simulink model "Buck_ZCS"  (R2024a)
settings: Solver=VariableStepAuto  StartTime=0.0  StopTime=10.0  RelTol=1e-3
values from neighbouring files (symbols this model uses):
  Cr = 10^(-6)    (= 1e-06)    [Parameters.m]
  Fs = 100*10^(3)    (= 100000)    [Parameters.m]
  Io = 1    [Parameters.m]
  Lr = 10*10^(-6)    (= 1e-05)    [Parameters.m]
  R = 7.69    [Parameters.m]
  Vin = 12    [Parameters.m]
  Wo = 1/sqrt(Lr*Cr)    [Parameters.m]
  Zo = sqrt(Lr/Cr)    [Parameters.m]
libraries: spsSeriesRLCBranchLib x6, spsCurrentMeasurementLib x2, spsDiodeLib x2, spsDCVoltageSourceLib x1, spsMosfetLib x1, spsVoltageMeasurementLib x1, sps_lib x1
settings Model: Creator=User  LastModifiedBy=User

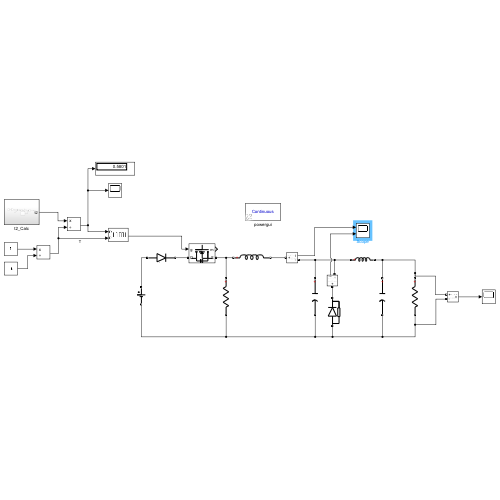
[thumbnail: Simulink's stored preview of the top-level diagram]
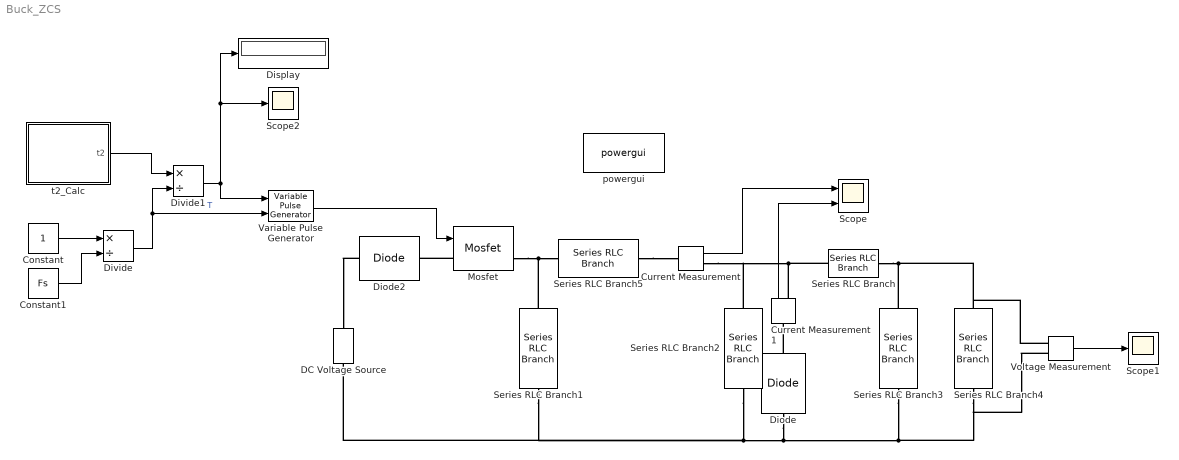
== system Buck_ZCS ==
  Constant : Constant
  Constant1 : Constant  Value=Fs
  Current Measurement : spsCurrentMeasurementLib/Current Measurement  PhasorSimulation=off  OutputType=Complex  PSBequivalent=0
  Current Measurement1 : spsCurrentMeasurementLib/Current Measurement  PhasorSimulation=off  OutputType=Complex  PSBequivalent=0
  DC Voltage Source : spsDCVoltageSourceLib/DC Voltage Source  Amplitude=Vin  Measurements=None
  Diode : spsDiodeLib/Diode  Ron=0.001  Lon=0  Vf=0.8  IC=0  UseSnubber=0  Rs=500  Cs=250e-9  Measurements=off
  Diode2 : spsDiodeLib/Diode  Ron=0.001  Lon=0  Vf=0.8  IC=0  UseSnubber=0  Rs=500  Cs=0  Measurements=off
  Display : Display
  Divide : Product  Inputs=*/
  Divide1 : Product  Inputs=*/
  Mosfet : spsMosfetLib/Mosfet  Ron=0.1  Lon=0  Rd=0.01  Vfd=0  IC=0  Rs=1e5  Cs=inf  Measurements=on
  Scope : Scope  NumInputPorts=2
  Scope1 : Scope
  Scope2 : Scope
  Series RLC Branch : spsSeriesRLCBranchLib/Series RLC Branch  LConnTagsString=__new0  RConnTagsString=__new0  BranchType=L  Resistance=1  Inductance=5e-3  SetiL0=off  InitialCurrent=0  Capacitance=1e-6  Setx0=off  InitialVoltage=0  Measurements=None
  Series RLC Branch1 : spsSeriesRLCBranchLib/Series RLC Branch  LConnTagsString=__new0  RConnTagsString=__new0  BranchType=R  Resistance=10000  Inductance=1e-3  SetiL0=off  InitialCurrent=0  Capacitance=1e-6  Setx0=off  InitialVoltage=0  Measurements=None
  Series RLC Branch2 : spsSeriesRLCBranchLib/Series RLC Branch  LConnTagsString=__new0  RConnTagsString=__new0  BranchType=C  Resistance=1  Inductance=1e-3  SetiL0=off  InitialCurrent=0  Capacitance=Cr  Setx0=off  InitialVoltage=0  Measurements=None
  Series RLC Branch3 : spsSeriesRLCBranchLib/Series RLC Branch  LConnTagsString=__new0  RConnTagsString=__new0  BranchType=C  Resistance=1  Inductance=1e-3  SetiL0=off  InitialCurrent=0  Capacitance=200e-6  Setx0=off  InitialVoltage=0  Measurements=None
  Series RLC Branch4 : spsSeriesRLCBranchLib/Series RLC Branch  LConnTagsString=__new0  RConnTagsString=__new0  BranchType=R  Resistance=R  Inductance=1e-3  SetiL0=off  InitialCurrent=0  Capacitance=1e-6  Setx0=off  InitialVoltage=0  Measurements=None
  Series RLC Branch5 : spsSeriesRLCBranchLib/Series RLC Branch  LConnTagsString=__new0  RConnTagsString=__new0  BranchType=L  Resistance=1  Inductance=Lr  SetiL0=off  InitialCurrent=0  Capacitance=1e-6  Setx0=off  InitialVoltage=0  Measurements=None
  Variable Pulse Generator : VariablePulseGenerator  SampleTime=0.1
  Voltage Measurement : spsVoltageMeasurementLib/Voltage Measurement  PhasorSimulation=off  OutputType=Complex  PSBequivalent=0
  powergui : sps_lib/powergui  Priority=1  SimulationMode=Continuous  SampleTime=50e-6  frequency=60  Iterations=50  frequencyindice=0  Pbase=100e6  ErrMax=1e-4  UnitsV=kV  UnitsW=MW  buscounter=0  FunctionMessages=off  echomessages=off  EnableUseOfTLC=off  CurrentSourceSwitches=off  DisableSnubberDevices=off  DisableRonSwitches=off  DisableVfSwitches=off  DisplayEquations=off  AutomaticDiscreteSolvers=off  SolverType=Tustin/Backward Euler (TBE)  Interpol=off  ExternalGateDelay=off  methode=off  Ts=100  x0status=blocks  SPID=on  SwTol=0  HookPort=off  NonlinearTolerance=1e-4  nMaxIteration=100  ContinueOnMaxIteration=off  RestoreLinks=warning  ResistiveCurrentMeasurement=off  Frange=[0:2:500]  Ylog=off  Xlog=on  ShowGrid=off  save=off  variable=ZData  structure=0  ZoomFFT=off  StartTime=0.0  cycles=1  DisplayStyle=1  fundamental=60  FreqAxis=off  MaxFrequency=1000  frequencyindicesteady=1  RmsSteady=1  display=off
  t2_Calc : Subsystem
  wires:
  Variable Pulse Generator/1 -> Mosfet/1
  Divide/1 -> Divide1/2, Variable Pulse Generator/2  "T"
  Constant/1 -> Divide/1
  Constant1/1 -> Divide/2
  Divide1/1 -> Variable Pulse Generator/1, Scope2/1, Display/1
  t2_Calc/1(t2) -> Divide1/1
  Current Measurement/1 -> Scope/1
  Voltage Measurement/1 -> Scope1/1
  Current Measurement1/1 -> Scope/2
  connections:
  Diode2/LConn1 -- DC Voltage Source/RConn1
  Series RLC Branch1/LConn1 -- Mosfet/RConn1 -- Series RLC Branch5/LConn1
  Series RLC Branch/LConn1 -- Series RLC Branch2/LConn1 -- Current Measurement/RConn1 -- Current Measurement1/RConn1
  Series RLC Branch3/LConn1 -- Series RLC Branch4/LConn1 -- Voltage Measurement/LConn1 -- Series RLC Branch/RConn1
  Series RLC Branch1/RConn1 -- DC Voltage Source/LConn1 -- Series RLC Branch2/RConn1 -- Diode/LConn1 -- Series RLC Branch4/RConn1 -- Voltage Measurement/LConn2 -- Series RLC Branch3/RConn1
  Series RLC Branch5/RConn1 -- Current Measurement/LConn1
  Mosfet/LConn1 -- Diode2/RConn1
  Diode/RConn1 -- Current Measurement1/LConn1

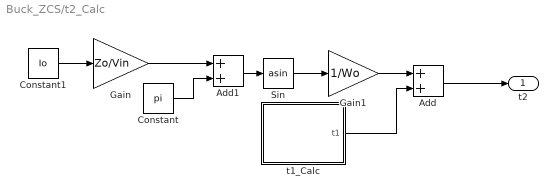
== system Buck_ZCS/t2_Calc ==
  Add : Sum
  Add1 : Sum
  Constant : Constant  Value=pi
  Constant1 : Constant  Value=Io
  Gain : Gain  Gain=Zo/Vin
  Gain1 : Gain  Gain=1/Wo
  Sin : Trigonometry  Operator=asin
  t1_Calc : Subsystem
  t2 : Outport
  wires:
  Add/1 -> t2/1
  Add1/1 -> Sin/1
  Constant/1 -> Add1/2
  Constant1/1 -> Gain/1
  Gain/1 -> Add1/1
  Sin/1 -> Gain1/1
  Gain1/1 -> Add/1
  t1_Calc/1(t1) -> Add/2

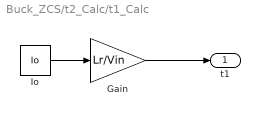
== system Buck_ZCS/t2_Calc/t1_Calc ==
  Gain : Gain  Gain=Lr/Vin
  Io : Constant  Value=Io
  t1 : Outport
  wires:
  Io/1 -> Gain/1
  Gain/1 -> t1/1
